simulink model "mc2_current_speed"  (R2023b)
settings: Solver=ode45  StartTime=0.0  StopTime=12  MaxStep=1e-5  RelTol=1e-3
libraries: spsDCVoltageSourceLib x1, spsUniversalBridgeLib x1, spsVoltageMeasurementLib x1, simulink x1, spspowerguiLib x1
settings Model: Creator=86189  LastModifiedBy=86189

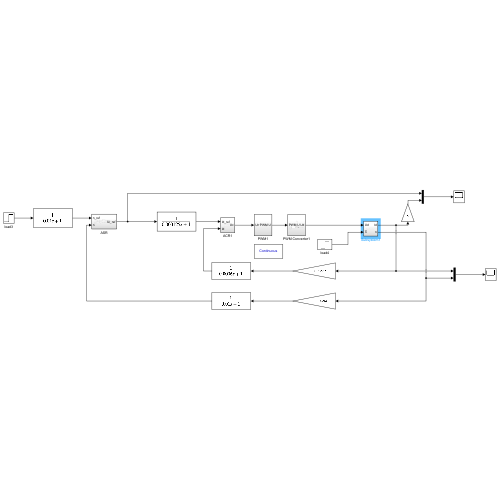
[thumbnail: Simulink's stored preview of the top-level diagram]
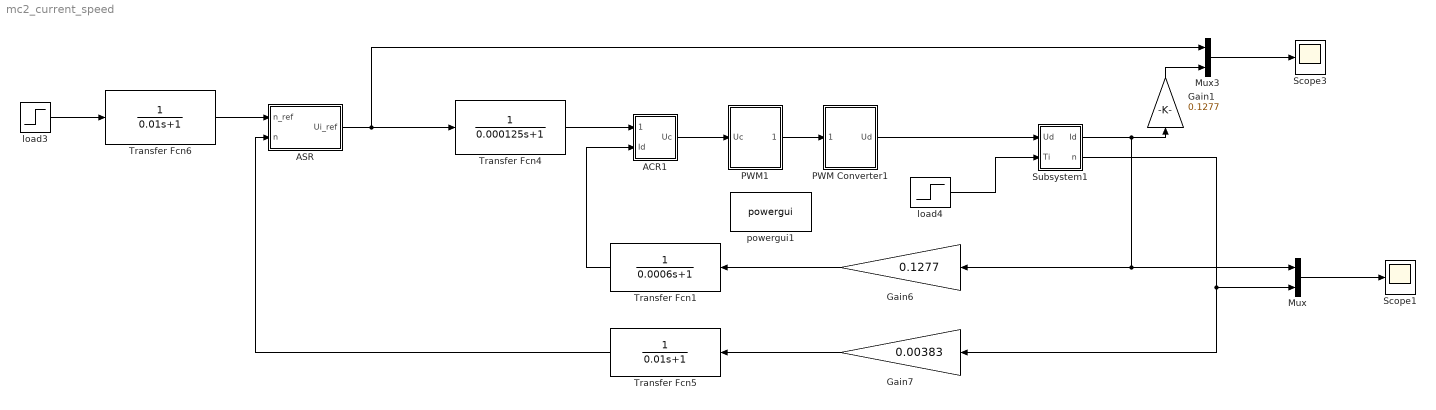
== system mc2_current_speed ==
  ACR1 : Subsystem
  ASR : Subsystem
  Gain1 : Gain  Gain=0.1277
  Gain6 : Gain  Gain=0.1277
  Gain7 : Gain  Gain=0.00383
  Mux : Mux  Inputs=2
  Mux3 : Mux  Inputs=2
  PWM Converter1 : Subsystem
  PWM1 : Subsystem
  Scope1 : Scope
  Scope3 : Scope
  Subsystem1 : Subsystem
  Transfer Fcn1 : TransferFcn  Denominator=[0.0006 1]
  Transfer Fcn4 : TransferFcn  Denominator=[0.000125 1]
  Transfer Fcn5 : TransferFcn  Denominator=[0.01 1]
  Transfer Fcn6 : TransferFcn  Denominator=[0.01 1]
  load3 : Step  Time=0  After=10  SampleTime=0
  load4 : Step  Time=0  After=0  SampleTime=0
  powergui1 : spspowerguiLib/powergui  Priority=1  SimulationMode=Continuous  SampleTime=50e-6  frequency=60  Iterations=50  frequencyindice=0  Pbase=100e6  ErrMax=1e-4  UnitsV=kV  UnitsW=MW  buscounter=0  FunctionMessages=off  echomessages=off  EnableUseOfTLC=off  CurrentSourceSwitches=off  DisableSnubberDevices=off  DisableRonSwitches=off  DisableVfSwitches=off  DisplayEquations=off  AutomaticDiscreteSolvers=off  SolverType=Tustin/Backward Euler (TBE)  Interpol=off  ExternalGateDelay=off  methode=off  Ts=100  x0status=blocks  SPID=on  SwTol=0  HookPort=off  NonlinearTolerance=1e-4  nMaxIteration=100  ContinueOnMaxIteration=off  RestoreLinks=warning  ResistiveCurrentMeasurement=off  Frange=[0:2:500]  Ylog=off  Xlog=on  ShowGrid=off  save=off  variable=ZData  structure=0  ZoomFFT=off  StartTime=0.0  cycles=1  DisplayStyle=1  fundamental=60  FreqAxis=off  MaxFrequency=1000  frequencyindicesteady=1  RmsSteady=1  display=off
  wires:
  Mux3/1 -> Scope3/1
  Gain1/1 -> Mux3/2
  Transfer Fcn5/1 -> ASR/2(n)
  PWM1/1(PWM U) -> PWM Converter1/1(PWM U)
  ACR1/1(Uc) -> PWM1/1(Uc)
  load3/1 -> Transfer Fcn6/1
  Transfer Fcn6/1 -> ASR/1(n_ref)
  ASR/1(Ui_ref) -> Mux3/1, Transfer Fcn4/1
  PWM Converter1/1(Ud) -> Subsystem1/1(Ud)
  Gain7/1 -> Transfer Fcn5/1
  Subsystem1/2(n) -> Mux/2, Gain7/1
  Transfer Fcn4/1 -> ACR1/1(Id_ref)
  Subsystem1/1(Id) -> Gain1/1, Mux/1, Gain6/1
  load4/1 -> Subsystem1/2(Ti)
  Gain6/1 -> Transfer Fcn1/1
  Transfer Fcn1/1 -> ACR1/2(Id)
  Mux/1 -> Scope1/1

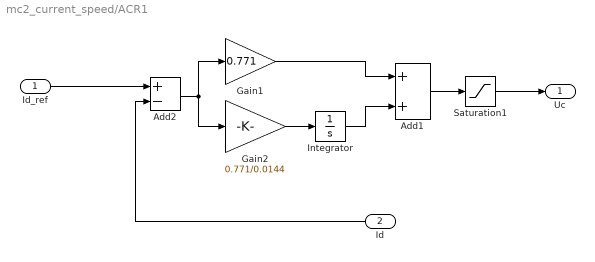
== system mc2_current_speed/ACR1 ==
  Id_ref : Inport
  Id : Inport  Port=2
  Add1 : Sum
  Add2 : Sum  Inputs=+-
  Gain1 : Gain  Gain=0.771
  Gain2 : Gain  Gain=0.771/0.0144
  Integrator : Integrator  LimitOutput=on  UpperSaturationLimit=5  LowerSaturationLimit=-5
  Saturation1 : Saturate  UpperLimit=5  LowerLimit=-5
  Uc : Outport
  wires:
  Gain2/1 -> Integrator/1
  Add1/1 -> Saturation1/1
  Integrator/1 -> Add1/2
  Add2/1 -> Gain2/1, Gain1/1
  Gain1/1 -> Add1/1
  Id/1 -> Add2/2
  Id_ref/1 -> Add2/1
  Saturation1/1 -> Uc/1

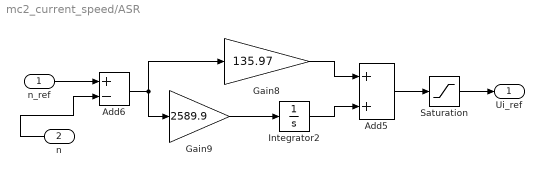
== system mc2_current_speed/ASR ==
  n_ref : Inport
  n : Inport  Port=2
  Add5 : Sum
  Add6 : Sum  Inputs=+-
  Gain8 : Gain  Gain=135.97
  Gain9 : Gain  Gain=2589.9
  Integrator2 : Integrator  LimitOutput=on  UpperSaturationLimit=5  LowerSaturationLimit=-5
  Saturation : Saturate  UpperLimit=5  LowerLimit=-5
  Ui_ref : Outport
  wires:
  Gain9/1 -> Integrator2/1
  n_ref/1 -> Add6/1
  Add6/1 -> Gain8/1, Gain9/1
  n/1 -> Add6/2
  Integrator2/1 -> Add5/2
  Gain8/1 -> Add5/1
  Add5/1 -> Saturation/1
  Saturation/1 -> Ui_ref/1

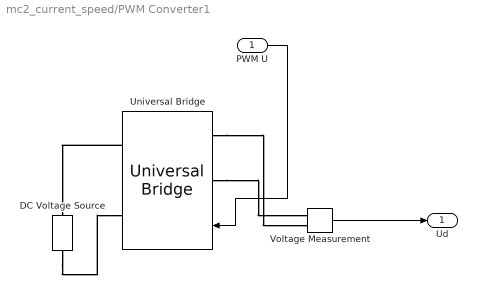
== system mc2_current_speed/PWM Converter1 ==
  PWM U : Inport
  DC Voltage Source : spsDCVoltageSourceLib/DC Voltage Source  Amplitude=538  Measurements=None
  Universal Bridge : spsUniversalBridgeLib/Universal Bridge  Arms=2  SnubberResistance=1e5  SnubberCapacitance=inf  Device=MOSFET / Diodes  Ron=1e-3  Lon=0  ForwardVoltages="[  0  0  ]"  ForwardVoltage=0  GTOparameters=[ 10e-6 , 20e-6 ]  IGBTparameters=[ 1e-6 , 2e-6 ]  Measurements=None  Measurements_2=None  converterType=Rectifier
  Voltage Measurement : spsVoltageMeasurementLib/Voltage Measurement  PhasorSimulation=off  OutputType=Complex  PSBequivalent=0
  Ud : Outport
  wires:
  PWM U/1 -> Universal Bridge/1
  Voltage Measurement/1 -> Ud/1
  connections:
  Universal Bridge/LConn2 -- Voltage Measurement/LConn2
  Universal Bridge/LConn1 -- Voltage Measurement/LConn1
  DC Voltage Source/RConn1 -- Universal Bridge/RConn1
  Universal Bridge/RConn2 -- DC Voltage Source/LConn1

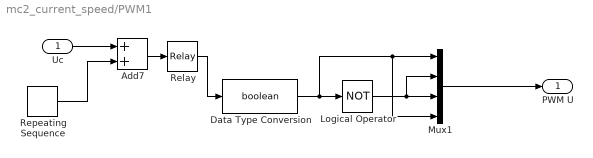
== system mc2_current_speed/PWM1 ==
  Uc : Inport
  Add7 : Sum
  Data Type Conversion : DataTypeConversion  OutDataTypeStr=boolean  SaturateOnIntegerOverflow=off  RndMeth=Floor
  Logical Operator : Logic  Operator=NOT  AllPortsSameDT=off  OutDataTypeStr=boolean
  Mux1 : Mux
      settings: DisplayOption=signals
  Relay : Relay  OnSwitchValue=0  OffSwitchValue=0
  Repeating Sequence : simulink/Sources/Repeating Sequence  rep_seq_t=[0 0.125e-3]  rep_seq_y=[-5 5]
  PWM U : Outport
  wires:
  Repeating Sequence/1 -> Add7/2
  Data Type Conversion/1 -> Mux1/4, Mux1/1, Logical Operator/1
  Logical Operator/1 -> Mux1/2, Mux1/3
  Add7/1 -> Relay/1
  Mux1/1 -> PWM U/1
  Relay/1 -> Data Type Conversion/1
  Uc/1 -> Add7/1

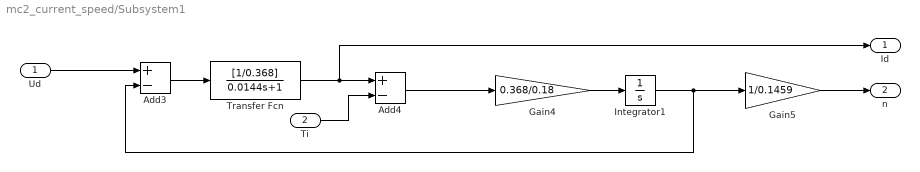
== system mc2_current_speed/Subsystem1 ==
  Ud : Inport
  Ti : Inport  Port=2
  Add3 : Sum  Inputs=+-
  Add4 : Sum  Inputs=+-
  Gain4 : Gain  Gain=0.368/0.18
  Gain5 : Gain  Gain=1/0.1459
  Integrator1 : Integrator
  Transfer Fcn : TransferFcn  Numerator=[1/0.368]  Denominator=[0.0144 1]
  Id : Outport
  n : Outport  Port=2
  wires:
  Add3/1 -> Transfer Fcn/1
  Transfer Fcn/1 -> Id/1, Add4/1
  Ud/1 -> Add3/1
  Add4/1 -> Gain4/1
  Integrator1/1 -> Add3/2, Gain5/1
  Gain4/1 -> Integrator1/1
  Gain5/1 -> n/1
  Ti/1 -> Add4/2
